simulink model "V4_3_1_Vorlage_Transistor"  (R2020a)
settings: Solver=VariableStepAuto  StartTime=0.0  StopTime=0.2  RelTol=1e-3
undefined symbols (not defined in the file): sigbuilder_block
libraries: fl_lib x16, nesl_utility x10, ee_lib x7, simulink x2
settings Model: Creator=schulte_n  LastModifiedBy=mkara
settings DataIOCC: ReturnWorkspaceOutputs=off
settings DebuggingCC: ArithmeticOperatorsInVariantConditions=warning
settings SFSimCC: SimUseLocalCustomCode=off  CustomCodeUndefinedFunction=UseInterfaceOnly
settings RTWCC: RTWUseLocalCustomCode=off

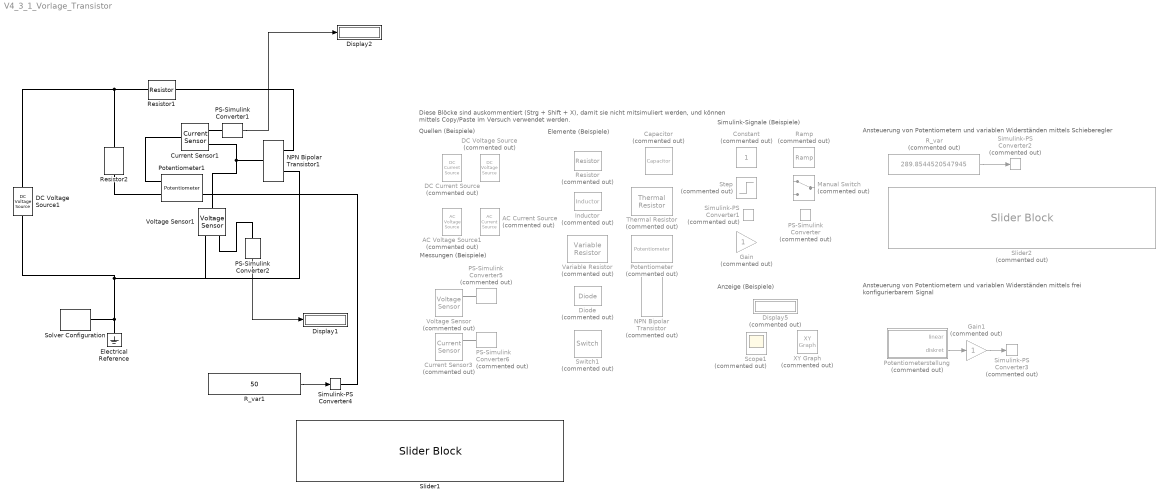
== system V4_3_1_Vorlage_Transistor ==
  note: Ansteuerung von Potentiometern und variablen Widerständen
      | mittels frei konfigurierbarem Signal
  note: Diese Blöcke sind auskommentiert (Strg + Shift + X), damit sie nicht mitsimuliert werden, und können mittels Copy/Paste im Versuch verwendet werden.
  note: Anzeige (Beispiele)
  note: Messungen (Beispiele)
  note: Elemente (Beispiele)
  note: Quellen (Beispiele)
  note: Simulink-Signale (Beispiele)
  note: Ansteuerung von Potentiometern und variablen Widerständen mittels Schieberegler
  AC Current Source : fl_lib/Electrical/Electrical Sources/AC Current Source  Commented=on  amp=1 A  shift=0 deg  frequency=60 Hz  omega=0 rad/s
      settings: SourceProductBaseCode=SS  InternalSimscapePortConfiguration="{\"Bottom\":[],\"Left\":[{\"id\":\"p\",\"label\":\"\",\"type\":\"foundation.electrical.electrical\"}],\"Right\":[{\"id\":\"n\",\"label\":\"\",\"type\":\"foundation.electrical.electrical\"}],\"Top\":[]}"
  AC Voltage Source1 : fl_lib/Electrical/Electrical Sources/AC Voltage Source  Commented=on  amp=1 V  shift=0 deg  frequency=60 Hz  omega=0 rad/s
  Capacitor : fl_lib/Electrical/Electrical Elements/Capacitor  Commented=on  c=1e-6 F  r=1e-6 Ohm  g=0 1/Ohm  i_specify=off  i_priority=None  i=0 A  i_nominal_specify=off  i_nominal_unit=A  i_nominal_value=1  v_specify=off  v_priority=None  v=0 V  v_nominal_specify=off  v_nominal_unit=V  v_nominal_value=1  vc_specify=off  vc_priority=High  vc=0 V  vc_nominal_specify=off  vc_nominal_unit=V  vc_nominal_value=1
  Constant : Constant  Commented=on
  Current Sensor1 : fl_lib/Electrical/Electrical Sensors/Current Sensor
  Current Sensor3 : fl_lib/Electrical/Electrical Sensors/Current Sensor  Commented=on
  DC Current Source : fl_lib/Electrical/Electrical Sources/DC Current Source  Commented=on  i0=1 A
      settings: SourceProductBaseCode=SS  InternalSimscapePortConfiguration="{\"Bottom\":[],\"Left\":[{\"id\":\"p\",\"label\":\"\",\"type\":\"foundation.electrical.electrical\"}],\"Right\":[{\"id\":\"n\",\"label\":\"\",\"type\":\"foundation.electrical.electrical\"}],\"Top\":[]}"
  DC Voltage Source : fl_lib/Electrical/Electrical Sources/DC Voltage Source  Commented=on  v0=1 V
  DC Voltage Source1 : fl_lib/Electrical/Electrical Sources/DC Voltage Source  v0=7 V
  Diode : fl_lib/Electrical/Electrical Elements/Diode  Commented=on  Vf=0.6 V  Ron=0.3 Ohm  Goff=1e-8 1/Ohm  i_specify=off  i_priority=None  i=0 A  i_nominal_specify=off  i_nominal_unit=A  i_nominal_value=1  v_specify=off  v_priority=None  v=0 V  v_nominal_specify=off  v_nominal_unit=V  v_nominal_value=1
  Display1 : Display
  Display2 : Display
  Display5 : Display  Commented=on
  Electrical Reference : fl_lib/Electrical/Electrical Elements/Electrical Reference
  Gain : Gain  Commented=on
  Gain1 : Gain  Commented=on
  Inductor : fl_lib/Electrical/Electrical Elements/Inductor  Commented=on  l=1e-6 H  r=0 Ohm  g=1e-9 1/Ohm  i_specify=off  i_priority=None  i=0 A  i_nominal_specify=off  i_nominal_unit=A  i_nominal_value=1  v_specify=off  v_priority=None  v=0 V  v_nominal_specify=off  v_nominal_unit=V  v_nominal_value=1  i_L_specify=off  i_L_priority=High  i_L=0 A  i_L_nominal_specify=off  i_L_nominal_unit=A  i_L_nominal_value=1
  Manual Switch : ManualSwitch  Commented=on
  NPN Bipolar Transistor : ee_lib/Semiconductors & Converters/NPN Bipolar Transistor  Commented=on  parameterization=1  prmDatasheet=1  prmEquCoeff=1  BF=100  IS=1e-14 A  VAF=200 V  hfe=100  hoe=50e-6 1/Ohm  Ic_h=1 mA  Vce_h=5 V  V1=0.55 V  I1=0.5 mA  BR=1  Tmeas=25 degC  RC=0.01 Ohm  RE=1e-4 Ohm  RB=1 Ohm  C_BC=5 pF  C_BE=5 pF  TF=0 us  TR=0 us  hfe_T2=125  XTB=0  V1_T2=0.45 V  I1_T2=0.5 mA  Tmeas2=125 degC  EG=1.11 eV  XTI=3  ec=1  TdeviceDatasheet=25 degC  TdeviceEquCoeff=25 degC  thermal_network_parameterization=ee.enum.thermalNetworkTopology.cauer  Rth=[0, 10] K/W  Rth_Foster=[4, 6] K/W  thermal_mass_parameterization=ee.enum.thermalNetwork.timeconstant  thermal_mass=[0, 1] J/K  thermal_mass_Foster=[1.5, 3] J/K  thermal_time_constant=[0, 10] s  thermal_time_constant_Foster=[6, 18] s  thermal_mass_initial_temperatures=[25, 25] degC
  NPN Bipolar Transistor1 : ee_lib/Semiconductors & Converters/NPN Bipolar Transistor  parameterization=1  prmDatasheet=1  prmEquCoeff=1  BF=100  IS=1e-14 A  VAF=200 V  hfe=100  hoe=50e-6 1/Ohm  Ic_h=1 mA  Vce_h=5 V  V1=0.55 V  I1=0.5 mA  BR=1  Tmeas=25 degC  RC=0.01 Ohm  RE=1e-4 Ohm  RB=1 Ohm  C_BC=5 pF  C_BE=5 pF  TF=0 us  TR=0 us  hfe_T2=125  XTB=0  V1_T2=0.45 V  I1_T2=0.5 mA  Tmeas2=125 degC  EG=1.11 eV  XTI=3  ec=1  TdeviceDatasheet=25 degC  TdeviceEquCoeff=25 degC  thermal_network_parameterization=ee.enum.thermalNetworkTopology.cauer  Rth=[0, 10] K/W  Rth_Foster=[4, 6] K/W  thermal_mass_parameterization=ee.enum.thermalNetwork.timeconstant  thermal_mass=[0, 1] J/K  thermal_mass_Foster=[1.5, 3] J/K  thermal_time_constant=[0, 10] s  thermal_time_constant_Foster=[6, 18] s  thermal_mass_initial_temperatures=[25, 25] degC
  PS-Simulink Converter : nesl_utility/PS-Simulink Converter  Commented=on  PhysicalDomain=network_engine_domain  SubClassName=ps_output  LeftPortType=input  RightPortType=output  PseudoPeriodic=off  Frequencies=[]  Unit=inherit  AffineConversion=off
  PS-Simulink Converter1 : nesl_utility/PS-Simulink Converter  PhysicalDomain=network_engine_domain  SubClassName=ps_output  LeftPortType=input  RightPortType=output  PseudoPeriodic=off  Frequencies=[]  Unit=1  AffineConversion=off
  PS-Simulink Converter2 : nesl_utility/PS-Simulink Converter  PhysicalDomain=network_engine_domain  SubClassName=ps_output  LeftPortType=input  RightPortType=output  PseudoPeriodic=off  Frequencies=[]  Unit=1  AffineConversion=off
  PS-Simulink Converter5 : nesl_utility/PS-Simulink Converter  Commented=on  PhysicalDomain=network_engine_domain  SubClassName=ps_output  LeftPortType=input  RightPortType=output  PseudoPeriodic=off  Frequencies=[]  Unit=1  AffineConversion=off
  PS-Simulink Converter6 : nesl_utility/PS-Simulink Converter  Commented=on  PhysicalDomain=network_engine_domain  SubClassName=ps_output  LeftPortType=input  RightPortType=output  PseudoPeriodic=off  Frequencies=[]  Unit=1  AffineConversion=off
  Potentiometer : ee_lib/Passive/Potentiometer  Commented=on  R0=1000 Ohm  Rw=1 Ohm  Rcenter=200 Ohm  xmin=0  xmax=1  Taper=1  Gradient=1
      settings: SourceProductBaseCode=PS  InternalSimscapePortConfiguration="{\"Bottom\":[],\"Left\":[{\"id\":\"pinL\",\"label\":\"L\",\"type\":\"foundation.electrical.electrical\"},{\"id\":\"W\",\"label\":\"W\",\"type\":\"foundation.electrical.electrical\"}],\"Right\":[{\"id\":\"pinR\",\"label\":\"R\",\"type\":\"foundation.electrical.electrical\"},{\"id\":\"x\",\"label\":\"x\",\"type\":\"input\"}],\"Top\":[]}"
  Potentiometer1 : ee_lib/Passive/Potentiometer  R0=50 kOhm  Rw=1 Ohm  Rcenter=200 Ohm  xmin=0  xmax=50  Taper=1  Gradient=1
      settings: SourceProductBaseCode=PS  InternalSimscapePortConfiguration="{\"Bottom\":[],\"Left\":[{\"id\":\"pinL\",\"label\":\"L\",\"type\":\"foundation.electrical.electrical\"},{\"id\":\"W\",\"label\":\"W\",\"type\":\"foundation.electrical.electrical\"}],\"Right\":[{\"id\":\"pinR\",\"label\":\"R\",\"type\":\"foundation.electrical.electrical\"},{\"id\":\"x\",\"label\":\"x\",\"type\":\"input\"}],\"Top\":[]}"
  Potentiometerstellung : Subsystem  Tag=STV Subsys  Commented=on  LoadFcn=sigbuilder_block('load');  StartFcn=sigbuilder_block('start');  StopFcn=sigbuilder_block('stop');  ClipboardFcn=sigbuilder_block('clipboard');  mask(Sigbuilder block){tuvar=[0:10]}
      mask help: Simulink:masks:SigbuilderBlock_MD
      mask init:
      | if ~strcmp(get_param(bdroot(gcbh),'SimulationStatus'),'stopped') tuvar = sigbuilder_block('maskInit'); end
      settings: CopyFcn=sigbuilder_block('copy');  DeleteFcn=sigbuilder_block('delete');  ModelCloseFcn=sigbuilder_block('modelClose');  PreSaveFcn=sigbuilder_block('preSave');  PauseFcn=sigbuilder_block('pause');  ContinueFcn=sigbuilder_block('continue');  NameChangeFcn=sigbuilder_block('namechange');  OpenFcn=sigbuilder_block('open',[462 201 550.5 399.75 ]);  CloseFcn=sigbuilder_block('close');
      mask Display: plot(0, 0, 100, 100,[2, 2, 32, 32, 2], [68, 8, 8, 68, 68],[32, 2], [38, 38], [32, 19, 2],[53, 60, 44], [32, 17, 17, 2],[16, 16, 31, 31]);txt = getActiveGroup(gcbh);text(2, 100, txt,'verticalAlignment', 'top');
  R_var : Constant  Commented=on  Value=289.8544520547945
  R_var1 : Constant  Value=50
  Ramp : simulink/Sources/Ramp  Commented=on  slope=1  start=0  InitialOutput=0
  Resistor : ee_lib/Passive/Resistor  Commented=on  R=1 Ohm  R_tol=5  enable_R_tol=0  tol_distribution=1  nSigma=4  enable_operating_limits=0  operating_limit_action=2  max_working_voltage=100 V  power_rating=1 W  enable_faults=0  fault_action=1  R_faulted=inf Ohm  enable_temporal_fault=0  t_fault=1 s  enable_behavioral_fault=0  max_permissible_current=1 A  t_fail_on_current=1 s  noise_mode=0  sample_time=1e-3 s  repeatability=1  auto_seed=3392865378  user_seed=0  Tdevice=25 degC  alpha=3.93e-3 1/K  Tmeas=25 degC  thermal_mass=100 J/K  power_derating_T1=70 degC  power_derating_T2=155 degC  operating_temperature_range_vec=[-50, 150] degC  temperature_specify=off  temperature_priority=High  temperature=298.15 K  temperature_nominal_specify=off  temperature_nominal_unit=K  temperature_nominal_value=1
  Resistor1 : ee_lib/Passive/Resistor  R=100 Ohm  R_tol=5  enable_R_tol=0  tol_distribution=1  nSigma=4  enable_operating_limits=0  operating_limit_action=2  max_working_voltage=100 V  power_rating=1 W  enable_faults=0  fault_action=1  R_faulted=inf Ohm  enable_temporal_fault=0  t_fault=1 s  enable_behavioral_fault=0  max_permissible_current=1 A  t_fail_on_current=1 s  noise_mode=0  sample_time=1e-3 s  repeatability=1  auto_seed=2061249901  user_seed=0  Tdevice=25 degC  alpha=3.93e-3 1/K  Tmeas=25 degC  thermal_mass=100 J/K  power_derating_T1=70 degC  power_derating_T2=155 degC  operating_temperature_range_vec=[-50, 150] degC  temperature_specify=off  temperature_priority=High  temperature=298.15 K  temperature_nominal_specify=off  temperature_nominal_unit=K  temperature_nominal_value=1
  Resistor2 : ee_lib/Passive/Resistor  R=1 kOhm  R_tol=5  enable_R_tol=0  tol_distribution=1  nSigma=4  enable_operating_limits=0  operating_limit_action=2  max_working_voltage=100 V  power_rating=1 W  enable_faults=0  fault_action=1  R_faulted=inf Ohm  enable_temporal_fault=0  t_fault=1 s  enable_behavioral_fault=0  max_permissible_current=1 A  t_fail_on_current=1 s  noise_mode=0  sample_time=1e-3 s  repeatability=1  auto_seed=3885752424  user_seed=0  Tdevice=25 degC  alpha=3.93e-3 1/K  Tmeas=25 degC  thermal_mass=100 J/K  power_derating_T1=70 degC  power_derating_T2=155 degC  operating_temperature_range_vec=[-50, 150] degC  temperature_specify=off  temperature_priority=High  temperature=298.15 K  temperature_nominal_specify=off  temperature_nominal_unit=K  temperature_nominal_value=1
  Scope1 : Scope  Commented=on
  Simulink-PS Converter1 : nesl_utility/Simulink-PS Converter  Commented=on  PhysicalDomain=network_engine_domain  SubClassName=ps_input  LeftPortType=input  RightPortType=output  PseudoPeriodic=off  Frequencies=[]  NoiseDistribution=none  NoiseParameters=[]  Unit=1  AffineConversion=off  FilteringAndDerivatives=provide  SimscapeFilterOrder=1  InputFilterTimeConstant=0.001  UdotUserProvided=0
  Simulink-PS Converter2 : nesl_utility/Simulink-PS Converter  Commented=on  PhysicalDomain=network_engine_domain  SubClassName=ps_input  LeftPortType=input  RightPortType=output  PseudoPeriodic=off  Frequencies=[]  NoiseDistribution=none  NoiseParameters=[]  Unit=1  AffineConversion=off  FilteringAndDerivatives=provide  SimscapeFilterOrder=1  InputFilterTimeConstant=0.001  UdotUserProvided=0
  Simulink-PS Converter3 : nesl_utility/Simulink-PS Converter  Commented=on  PhysicalDomain=network_engine_domain  SubClassName=ps_input  LeftPortType=input  RightPortType=output  PseudoPeriodic=off  Frequencies=[]  NoiseDistribution=none  NoiseParameters=[]  Unit=1  AffineConversion=off  FilteringAndDerivatives=provide  SimscapeFilterOrder=1  InputFilterTimeConstant=0.001  UdotUserProvided=0
  Simulink-PS Converter4 : nesl_utility/Simulink-PS Converter  PhysicalDomain=network_engine_domain  SubClassName=ps_input  LeftPortType=input  RightPortType=output  PseudoPeriodic=off  Frequencies=[]  NoiseDistribution=none  NoiseParameters=[]  Unit=1  AffineConversion=off  FilteringAndDerivatives=provide  SimscapeFilterOrder=1  InputFilterTimeConstant=0.001  UdotUserProvided=0
  Slider1 : SliderBlock  ScaleMax=50  TickInterval=1
  Slider2 : SliderBlock  Commented=on  ScaleMax=1000  TickInterval=100
  Solver Configuration : nesl_utility/Solver Configuration  PhysicalDomain=network_engine_domain  SubClassName=solver  LeftPortType=input  RightPortType=generic  Tones=[]  Harmonics=[]  SimulateNoise=off  Profile=off  UseLocalSampling=off  EnableSwitchedLinearOptims=on  FrequencyDomain=off  UseCCode=off  RelTol=0.001  AbsTol=1e-06  MinStep=1e-09  ToWorkspace=off  RevertToSquareIcSolve=off  NumHomotopyIterations=100  PhasorMode=off  PhasorModeNumHarmonics=1  DoDC=off  ResidualTolerance=1e-09  UseLocalSolver=off  LocalSolverChoice=NE_BACKWARD_EULER_ADVANCER  LocalSolverSampleTime=0.001  DoFixedCost=off  MaxNonlinIter=3  MaxModeIter=2  LinearAlgebra=Sparse  EquationFormulation=NE_TIME_EF  DelaysMemoryBudget=1024  AutomaticFiltering=on  FilteringTimeConstant=0.001  PartitionStorageMethod=AS_NEEDED  PartitionMemoryBudget=1024  PartitionMethod=FAST
  Step : Step  Commented=on  SampleTime=0
  Switch1 : fl_lib/Electrical/Electrical Elements/Switch  Commented=on  R_closed=0.01 Ohm  G_open=1e-8 1/Ohm  Threshold=0  i_specify=off  i_priority=None  i=0 A  i_nominal_specify=off  i_nominal_unit=A  i_nominal_value=1  v_specify=off  v_priority=None  v=0 V  v_nominal_specify=off  v_nominal_unit=V  v_nominal_value=1
  Thermal Resistor : fl_lib/Electrical/Electrical Elements/Thermal Resistor  Commented=on  R0=1 Ohm  T0=298.15 K  alpha=50e-6 1/K  tc=10 s  K_d=1e-3 W/K  T_specify=off  T_priority=High  T=300 K  T_nominal_specify=off  T_nominal_unit=K  T_nominal_value=1
      settings: SourceProductBaseCode=SS  InternalSimscapePortConfiguration="{\"Bottom\":[],\"Left\":[{\"id\":\"H\",\"label\":\"H\",\"type\":\"foundation.thermal.thermal\"},{\"id\":\"p\",\"label\":\"+\",\"type\":\"foundation.electrical.electrical\"}],\"Right\":[{\"id\":\"n\",\"label\":\"-\",\"type\":\"foundation.electrical.electrical\"}],\"Top\":[]}"
  Variable Resistor : fl_lib/Electrical/Electrical Elements/Variable Resistor  Commented=on  Rmin=0 Ohm  i_specify=off  i_priority=None  i=0 A  i_nominal_specify=off  i_nominal_unit=A  i_nominal_value=1  v_specify=off  v_priority=None  v=0 V  v_nominal_specify=off  v_nominal_unit=V  v_nominal_value=1
  Voltage Sensor : fl_lib/Electrical/Electrical Sensors/Voltage Sensor  Commented=on
  Voltage Sensor1 : fl_lib/Electrical/Electrical Sensors/Voltage Sensor
  XY Graph : simulink/Sinks/XY Graph  Commented=on  xmin=-1  xmax=1  ymin=-1  ymax=1  st=-1
  wires:
  R_var/1 -> Simulink-PS Converter2/1
  Potentiometerstellung/2(diskret) -> Gain1/1
  Gain1/1 -> Simulink-PS Converter3/1
  R_var1/1 -> Simulink-PS Converter4/1
  PS-Simulink Converter1/1 -> Display2/1
  PS-Simulink Converter2/1 -> Display1/1
  connections:
  Solver Configuration/RConn1 -- Voltage Sensor1/RConn2 -- NPN Bipolar Transistor1/RConn2 -- DC Voltage Source1/RConn1 -- Electrical Reference/LConn1
  PS-Simulink Converter5/LConn1 -- Voltage Sensor/RConn1
  PS-Simulink Converter6/LConn1 -- Current Sensor3/RConn1
  DC Voltage Source1/LConn1 -- Resistor2/LConn1 -- Resistor1/LConn1
  Resistor1/RConn1 -- NPN Bipolar Transistor1/RConn1
  Potentiometer1/LConn2 -- Resistor2/RConn1
  Simulink-PS Converter4/RConn1 -- Potentiometer1/RConn2
  PS-Simulink Converter1/LConn1 -- Current Sensor1/RConn1
  Current Sensor1/RConn2 -- Voltage Sensor1/LConn1 -- NPN Bipolar Transistor1/LConn1
  Potentiometer1/LConn1 -- Current Sensor1/LConn1
  PS-Simulink Converter2/LConn1 -- Voltage Sensor1/RConn1

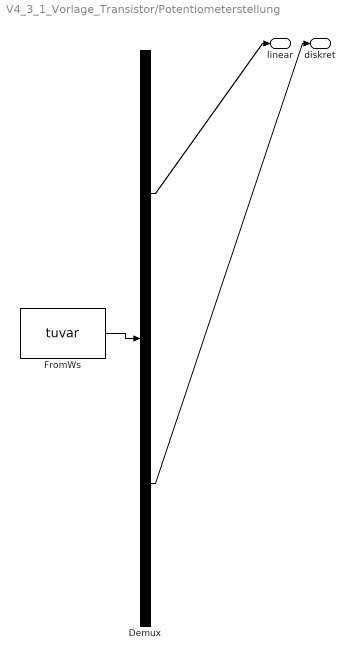
== system V4_3_1_Vorlage_Transistor/Potentiometerstellung ==
  Demux : Demux  Tag=STV Demux  Outputs=2
      settings: DisplayOption=none
  FromWs : FromWorkspace  Tag=STV FromWs  VariableName=tuvar
      SigBuilderData=|
      | common.afterFinalStr = 'Extrapolate'
      | common.sampleTime = 0
      | dataSet.timeRange = [0 11]
      | dataSet.name = 'Group 1'
      | sbobj.Groups.Name = 'Group 1'
      | sbobj.Groups.Signals(1).Name = 'linear'
      | sbobj.Groups.Signals(1).XData = [0 1 2 3 4 5 6 7 8 9 10 11]
      | sbobj.Groups.Signals(1).YData = [0 1 2 3 4 5 6 7 8 9 10 10]
      | sbobj.Groups.Signals(2).Name = 'diskret'
      | sbobj.Groups.Signals(2).XData = [0 1 1 2 2 3 3 4 4 5 5 6 6 7 7 8 8 9 9 10 10 11]
      | sbobj.Groups.Signals(2).YData = [0 0 1 1 2 2 3 3 4 4 5 5 6 6 7 7 8 8 9 9 10 10]
      | sbobj.Groups.TimeRange = [0 11]
  linear : Outport  Tag=STV Outport
  diskret : Outport  Tag=STV Outport  Port=2
  wires:
  FromWs/1 -> Demux/1
  Demux/1 -> linear/1
  Demux/2 -> diskret/1
